simulink model "DEM_testbench_DACerrors"  (Simulink 8.1)
settings: Solver=FixedStepDiscrete  StartTime=0.0  StopTime=60e-3  RelTol=1e-3
values from neighbouring files (symbols this model uses):
  dem_dcin = 1    [init_DAC_3ele.m]    (also in init_DAC_8ele.m)
  dem_select = 4    [init_DAC_3ele.m]    (also in init_DAC_8ele.m)
  dem_sinamp = 2    [init_DAC_3ele.m]    (also in init_DAC_8ele.m = 7)
  dem_sinfreq = 4882.8125    [init_DAC_3ele.m]    (also in init_DAC_8ele.m)
undefined symbols (not defined in the file or in its folder): DACctrl, Fs
libraries: simulink x4, dspsigops x3, dspsrcs4 x2
settings Model: Creator=amyles  LastModifiedBy=amyles
settings DataIOCC: MaxDataPoints=50000
settings DebuggingCC: ParameterPrecisionLossMsg=none  StrictBusMsg=Warning
settings SFSimCC: SimParseCustomCode=off

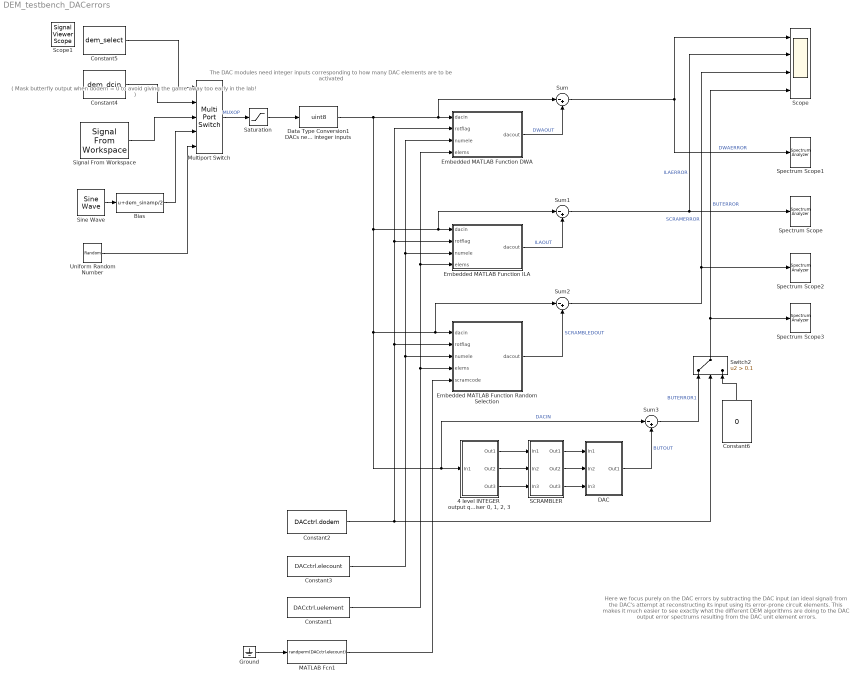
== system DEM_testbench_DACerrors ==
  note: The DAC modules need integer
      | inputs corresponding to how many
      | DAC elements are to be activated
  note: Here we focus purely on the DAC errors by
      | subtracting the DAC input (an ideal signal) from the
      | DAC's attempt at reconstructing its input using its
      | error-prone circuit elements.
      |
      | This makes it much easier to see exactly what the different
      | DEM algorithms are doing to the DAC output error
      | spectrums resulting from the DAC unit element errors.
  note: ( Mask butterfly output when dodem = 0
      | to avoid giving the game away too early
      | in the lab! )
  "4 level INTEGER  output quantiser 0, 1, 2, 3" : Subsystem
  Bias : Bias  Bias=dem_sinamp/2
  Constant1 : Constant  Value=DACctrl.uelement  SampleTime=1/Fs
  Constant2 : Constant  Value=DACctrl.dodem  SampleTime=1/Fs
  Constant3 : Constant  Value=DACctrl.elecount  SampleTime=1/Fs
  Constant4 : Constant  Value=dem_dcin  SampleTime=1/Fs
  Constant5 : Constant  Value=dem_select  SampleTime=1/Fs
  Constant6 : Constant  Value=0  SampleTime=1/Fs
  DAC : Subsystem
  Data Type Conversion1 DACs need integer inputs : DataTypeConversion  OutDataTypeStr=uint8  RndMeth=Nearest
  Embedded MATLAB Function DWA : MATLAB Function  TreatAsAtomicUnit=on
  Embedded MATLAB Function ILA : MATLAB Function  TreatAsAtomicUnit=on
  Embedded MATLAB Function Random Selection : MATLAB Function  TreatAsAtomicUnit=on
  Ground : Ground
  MATLAB Fcn1 : MATLABFcn  MATLABFcn=randperm(DACctrl.elecount)  SampleTime=1/Fs
  Multiport Switch : MultiPortSwitch  Inputs=4
  SCRAMBLER : Subsystem
  Saturation : Saturate  UpperLimit=DACctrl.elecount  LowerLimit=0
  Scope : Scope  NumInputPorts=4
      settings: YMin=-0.04~-5~-5~-5  YMax=0.04~5~5~5
  Signal From Workspace : dspsrcs4/Signal From Workspace  X=[1 1 2]  Ts=1/Fs  nsamps=1  OutputAfterFinalValue=Cyclic repetition  ignoreOrWarnInputAndFrameLengths=off
  Sine Wave : dspsrcs4/Sine Wave  Amplitude=dem_sinamp/2  Frequency=dem_sinfreq  Phase=0  SampleMode=Discrete  OutComplex=Real  CompMethod=Trigonometric fcn  TableSize=Speed  SampleTime=1/Fs  SamplesPerFrame=1  ResetState=Restart at time zero  dataType=double  wordLen=16  udDataType=sfix(16)  fracBitsMode=Best precision  numFracBits=15  OutDataTypeStr=double  LastOutDataTypeStr=double
  Spectrum Scope{,1..3} (4 alike) : SpectrumAnalyzer
      settings: CopyFcn=scopeextensions.ScopeBlock.callback(gcbh, 'onBlockCopy', gcbh);  DeleteFcn=scopeextensions.ScopeBlock.callback(gcbh, 'onBlockDelete');  PreSaveFcn=scopeextensions.ScopeBlock.callback(gcbh, 'onModelSave');  NameChangeFcn=scopeextensions.ScopeBlock.callback(gcbh, 'onBlockRename');  CloseFcn=scopeextensions.ScopeBlock.callback(gcbh, 'onBlockClose');  PreDeleteFcn=scopeextensions.ScopeBlock.callback(gcbh, 'onBlockPreDelete');
  Sum{,1..3} (4 alike) : Sum  Inputs=|-+
  Switch2 : Switch  Criteria=u2 > Threshold  Threshold=0.1
  Uniform Random Number : UniformRandomNumber  Minimum=0  Maximum=DACctrl.elecount  SampleTime=1/Fs
  Scope1 : SignalViewerScope  IOType=viewer  NumInputPorts=2  ZoomMode=xonly  RefreshTime=0.035000
      settings: YMin=0~0  YMax=3~3
  wires:
  Constant5/1 -> Multiport Switch/1
  Signal From Workspace/1 -> Multiport Switch/3
  Sine Wave/1 -> Bias/1
  Multiport Switch/1 -> Saturation/1  "MUXOP"
  Data Type Conversion1 DACs need integer inputs/1 -> Embedded MATLAB Function ILA/1(dacin), Sum1/1, Embedded MATLAB Function Random Selection/1(dacin), Sum2/1, Sum3/1, "4 level INTEGER  output quantiser 0, 1, 2, 3"/1(In1), Embedded MATLAB Function DWA/1(dacin), Sum/1  "DACIN"
  Saturation/1 -> Data Type Conversion1 DACs need integer inputs/1
  Bias/1 -> Multiport Switch/4
  Uniform Random Number/1 -> Multiport Switch/5
  Constant4/1 -> Multiport Switch/2
  Constant2/1 -> Embedded MATLAB Function DWA/2(rotflag), Embedded MATLAB Function ILA/2(rotflag), Embedded MATLAB Function Random Selection/2(rotflag), Switch2/2
  Constant3/1 -> Embedded MATLAB Function DWA/3(numele), Embedded MATLAB Function ILA/3(numele), Embedded MATLAB Function Random Selection/3(numele)
  Constant1/1 -> Embedded MATLAB Function DWA/4(elems), Embedded MATLAB Function ILA/4(elems), Embedded MATLAB Function Random Selection/4(elems)
  Embedded MATLAB Function DWA/1(dacout) -> Sum/2  "DWAOUT"
  Embedded MATLAB Function ILA/1(dacout) -> Sum1/2  "ILAOUT"
  Embedded MATLAB Function Random Selection/1(dacout) -> Sum2/2  "SCRAMBLEDOUT"
  Sum/1 -> Scope/1, Spectrum Scope1/1  "DWAERROR"
  Sum1/1 -> Scope/2, Spectrum Scope/1  "ILAERROR"
  Sum2/1 -> Spectrum Scope2/1, Scope/3  "SCRAMERROR"
  MATLAB Fcn1/1 -> Embedded MATLAB Function Random Selection/5(scramcode)
  Ground/1 -> MATLAB Fcn1/1
  "4 level INTEGER  output quantiser 0, 1, 2, 3"/1(Out1) -> SCRAMBLER/1(In1)
  "4 level INTEGER  output quantiser 0, 1, 2, 3"/2(Out2) -> SCRAMBLER/2(In2)
  "4 level INTEGER  output quantiser 0, 1, 2, 3"/3(Out3) -> SCRAMBLER/3(In3)
  SCRAMBLER/1(Out1) -> DAC/1(In1)
  SCRAMBLER/2(Out2) -> DAC/2(In2)
  SCRAMBLER/3(Out3) -> DAC/3(In3)
  DAC/1(Out1) -> Sum3/2  "BUTOUT"
  Switch2/1 -> Spectrum Scope3/1, Scope/4  "BUTERROR"
  Constant6/1 -> Switch2/3
  Sum3/1 -> Switch2/1  "BUTERROR1"

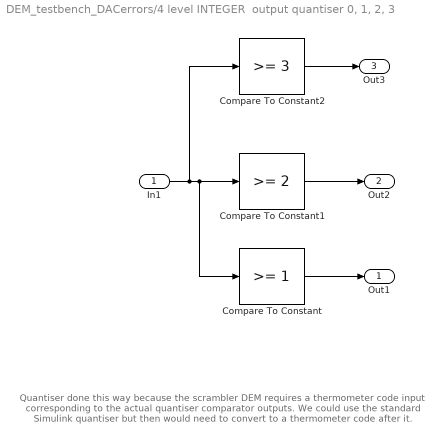
== system DEM_testbench_DACerrors/4 level INTEGER  output quantiser 0, 1, 2, 3 ==
  note: Quantiser done this way because the scrambler DEM
      | requires a thermometer code input corresponding to
      | the actual quantiser comparator outputs. We could use the
      | standard Simulink quantiser but then would need to convert
      | to a thermometer code after it.
  In1 : Inport
  Compare To Constant : simulink/Logic and Bit Operations/Compare To Constant  relop=>=  const=1  OutDataTypeStr=uint8
  Compare To Constant1 : simulink/Logic and Bit Operations/Compare To Constant  relop=>=  const=2  OutDataTypeStr=uint8
  Compare To Constant2 : simulink/Logic and Bit Operations/Compare To Constant  relop=>=  const=3  OutDataTypeStr=uint8
  Out1 : Outport
  Out2 : Outport  Port=2
  Out3 : Outport  Port=3
  wires:
  Compare To Constant2/1 -> Out3/1
  Compare To Constant1/1 -> Out2/1
  Compare To Constant/1 -> Out1/1
  In1/1 -> Compare To Constant2/1, Compare To Constant1/1, Compare To Constant/1

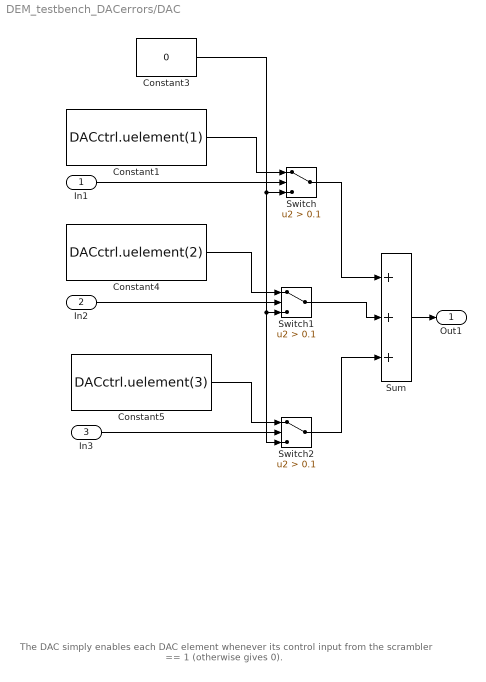
== system DEM_testbench_DACerrors/DAC ==
  note: The DAC simply enables each DAC element whenever its control
      | input from the scrambler == 1 (otherwise gives 0).
  In1 : Inport
  In2 : Inport  Port=2
  In3 : Inport  Port=3
  Constant1 : Constant  Value=DACctrl.uelement(1)  SampleTime=1/Fs
  Constant3 : Constant  Value=0  SampleTime=1/Fs
  Constant4 : Constant  Value=DACctrl.uelement(2)  SampleTime=1/Fs
  Constant5 : Constant  Value=DACctrl.uelement(3)  SampleTime=1/Fs
  Sum : Sum  Inputs=+++
  Switch : Switch  Criteria=u2 > Threshold  Threshold=0.1
  Switch1 : Switch  Criteria=u2 > Threshold  Threshold=0.1
  Switch2 : Switch  Criteria=u2 > Threshold  Threshold=0.1
  Out1 : Outport
  wires:
  Constant5/1 -> Switch2/1
  Constant4/1 -> Switch1/1
  Constant1/1 -> Switch/1
  Constant3/1 -> Switch2/3, Switch1/3, Switch/3
  In3/1 -> Switch2/2
  Sum/1 -> Out1/1
  In2/1 -> Switch1/2
  In1/1 -> Switch/2
  Switch2/1 -> Sum/3
  Switch1/1 -> Sum/2
  Switch/1 -> Sum/1

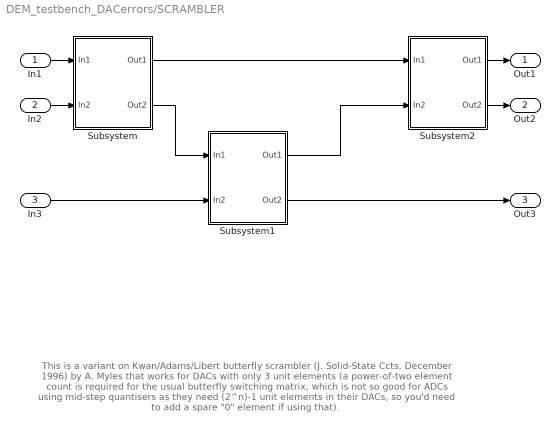
== system DEM_testbench_DACerrors/SCRAMBLER ==
  note: This is a variant on
      |
      | Kwan/Adams/Libert butterfly scrambler
      | (J. Solid-State Ccts. December 1996)
      |
      | by A. Myles that works for DACs with only 3 unit elements
      | (a power-of-two element count is required for the usual
      | butterfly switching matrix, which is not so good for
      | ADCs using mid-step quantisers as they need
      | (2^n)-1 unit elements in their DACs, so you'd need to
      | add a spare "0" element if using that).
  In1 : Inport
  In2 : Inport  Port=2
  In3 : Inport  Port=3
  Subsystem : Subsystem
  Subsystem1 : Subsystem
      settings: AttributesFormatString=Non-standard\nswitching block
  Subsystem2 : Subsystem
  Out1 : Outport
  Out2 : Outport  Port=2
  Out3 : Outport  Port=3
  wires:
  Subsystem1/1(Out1) -> Subsystem2/2(In2)
  Subsystem/2(Out2) -> Subsystem1/1(In1)
  Subsystem1/2(Out2) -> Out3/1
  In3/1 -> Subsystem1/2(In2)
  Subsystem2/2(Out2) -> Out2/1
  In2/1 -> Subsystem/2(In2)
  Subsystem2/1(Out1) -> Out1/1
  In1/1 -> Subsystem/1(In1)
  Subsystem/1(Out1) -> Subsystem2/1(In1)

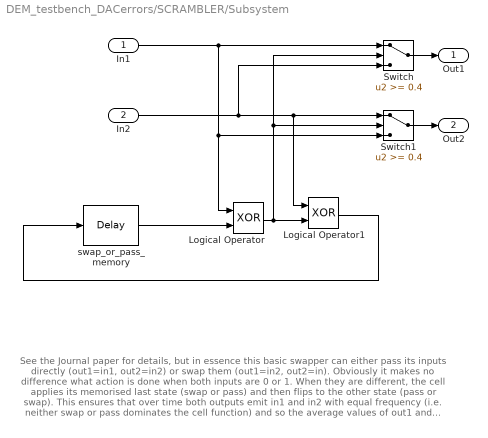
== system DEM_testbench_DACerrors/SCRAMBLER/Subsystem ==
  note: See the Journal paper for details, but in essence this basic swapper
      | can either pass its inputs directly (out1=in1, out2=in2) or swap
      | them (out1=in2, out2=in). Obviously it makes no difference what
      | action is done when both inputs are 0 or 1. When they are different,
      | the cell applies its memorised last state (swap or pass) and then flips
      | to the other state (pass or swap). This ensures that over time
      | both outputs emit in1 and in2 with equal frequency (i.e. neither
      | swap or pass dominates the cell function) and so the average values
      | of out1 and out2 are both (in1+in2)/2.
  In1 : Inport
  In2 : Inport  Port=2
  Logical Operator : Logic  Operator=XOR  AllPortsSameDT=off  OutDataTypeStr=boolean
  Logical Operator1 : Logic  Operator=XOR  AllPortsSameDT=off  OutDataTypeStr=boolean
  Switch : Switch  Threshold=0.4
  Switch1 : Switch  Threshold=0.4
  swap_or_pass_memory : dspsigops/Delay  InputProcessing=Columns as channels (frame based)  dly_unit=Samples  delay=1  ic_detail=off  dif_ic_for_ch=off  dif_ic_for_dly=off  ic=0  reset_popup=None
  Out1 : Outport
  Out2 : Outport  Port=2
  wires:
  Switch1/1 -> Out2/1
  Switch/1 -> Out1/1
  swap_or_pass_memory/1 -> Logical Operator/2
  Logical Operator1/1 -> swap_or_pass_memory/1
  Logical Operator/1 -> Logical Operator1/2, Switch1/2, Switch/2
  In2/1 -> Switch/3, Switch1/1, Logical Operator1/1
  In1/1 -> Switch/1, Switch1/3, Logical Operator/1

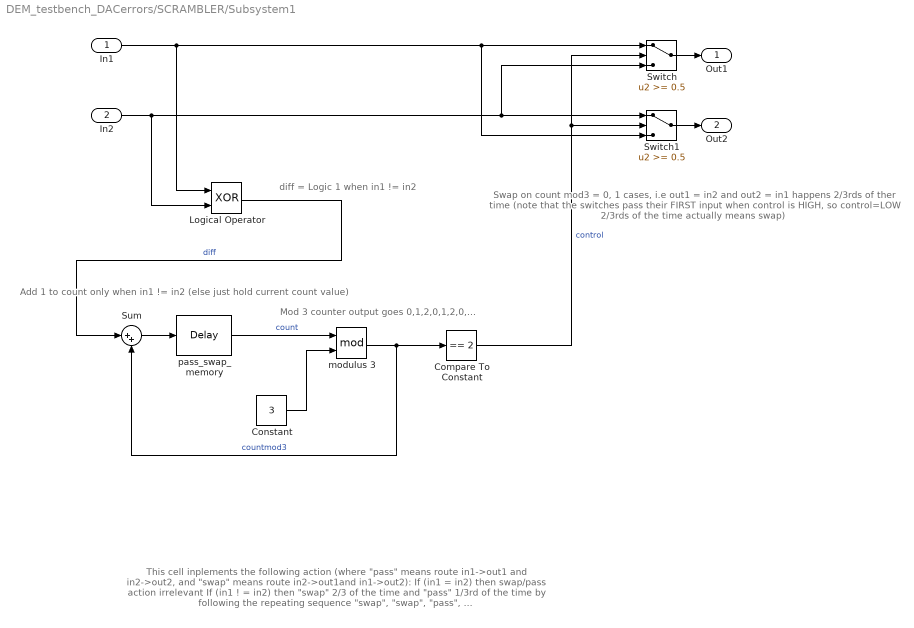
== system DEM_testbench_DACerrors/SCRAMBLER/Subsystem1 ==
  note: Swap on count mod3 = 0, 1 cases,
      | i.e out1 = in2 and out2 = in1
      | happens 2/3rds of ther time
      | (note that the switches pass
      | their FIRST input when control
      | is HIGH, so control=LOW 2/3rds
      | of the time actually means swap)
  note: Mod 3 counter output goes 0,1,2,0,1,2,0,...
  note: diff = Logic 1 when in1 != in2
  note: This cell inplements the following action
      | (where "pass" means route in1->out1 and in2->out2,
      | and "swap" means route in2->out1and in1->out2):
      |
      | If (in1 = in2) then swap/pass action irrelevant
      |
      | If (in1 ! = in2) then "swap" 2/3 of the time and "pass"
      | 1/3rd of the time by following the repeating sequence
      | "swap", "swap", "pass", ...
  note: Add 1 to count only when in1 != in2
      | (else just hold current count value)
  In1 : Inport
  In2 : Inport  Port=2
  Compare To Constant : simulink/Logic and Bit Operations/Compare To Constant  relop===  const=2  OutDataTypeStr=boolean
  Constant : Constant  Value=3
  Logical Operator : Logic  Operator=XOR  AllPortsSameDT=off  OutDataTypeStr=boolean
  Sum : Sum  Inputs=|++
  Switch : Switch  Threshold=0.5
  Switch1 : Switch  Threshold=0.5
  modulus 3 : Math  Operator=mod  SaturateOnIntegerOverflow=on
  pass_swap_memory : dspsigops/Delay  InputProcessing=Columns as channels (frame based)  dly_unit=Samples  delay=1  ic_detail=off  dif_ic_for_ch=off  dif_ic_for_dly=off  ic=0  reset_popup=None
  Out1 : Outport
  Out2 : Outport  Port=2
  wires:
  Compare To Constant/1 -> Switch/2, Switch1/2  "control"
  Sum/1 -> pass_swap_memory/1
  pass_swap_memory/1 -> modulus 3/1  "count"
  modulus 3/1 -> Sum/2, Compare To Constant/1  "countmod3"
  Constant/1 -> modulus 3/2
  Logical Operator/1 -> Sum/1  "diff"
  In1/1 -> Logical Operator/1, Switch1/3, Switch/1
  In2/1 -> Logical Operator/2, Switch1/1, Switch/3
  Switch/1 -> Out1/1
  Switch1/1 -> Out2/1

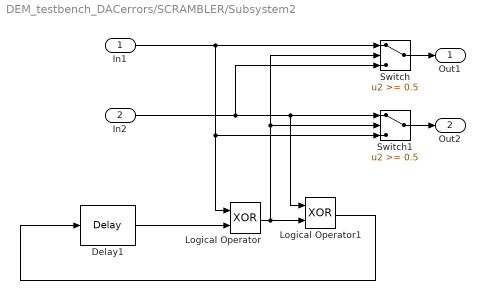
== system DEM_testbench_DACerrors/SCRAMBLER/Subsystem2 ==
  In1 : Inport
  In2 : Inport  Port=2
  Delay1 : dspsigops/Delay  InputProcessing=Columns as channels (frame based)  dly_unit=Samples  delay=1  ic_detail=off  dif_ic_for_ch=off  dif_ic_for_dly=off  ic=0  reset_popup=None
  Logical Operator : Logic  Operator=XOR  AllPortsSameDT=off  OutDataTypeStr=boolean
  Logical Operator1 : Logic  Operator=XOR  AllPortsSameDT=off  OutDataTypeStr=boolean
  Switch : Switch  Threshold=0.5
  Switch1 : Switch  Threshold=0.5
  Out1 : Outport
  Out2 : Outport  Port=2
  wires:
  In1/1 -> Logical Operator/1, Switch1/3, Switch/1
  In2/1 -> Logical Operator1/1, Switch1/1, Switch/3
  Logical Operator/1 -> Switch/2, Switch1/2, Logical Operator1/2
  Logical Operator1/1 -> Delay1/1
  Delay1/1 -> Logical Operator/2
  Switch/1 -> Out1/1
  Switch1/1 -> Out2/1

== matlab function Embedded MATLAB Function ILA ==
  data: dacin input double; dacout output double; rotflag input double; numele input double; elems input double
function dacout = DAC(dacin, rotflag, numele, elems)
%#eml

% This function assumes a MATLAB workspace structures exists called
% DACctrl with contents:
%
% DACctrl.dodem = DEM enable flag, 0 = no ILA, 1 = apply ILA
% DACctrl.elecount = number fo unit elements in the DAC
% DACctrl.uelement(1) = size of first unit element
% ...
% DACctrl.uelement(elecount) = size of last unit element

% ------------------ Begin Copyright notice -----------------------------
%
% COPYRIGHT AND PROPERTY OF DIALOG SEMICONDUCTOR, 2012.
%
% THIS COPYRIGHT NOTICE MUST NOT BE REMOVED OR MODIFIED.
%
% Commerical use is not permitted.
%
% Installation on systems available for use in any way by commercial users
% is not permitted.
%
% Permission for use is granted by Dialog Semiconductor only for the
% purposes of teaching or studying course ELEE11080/PGEE11110 "Sigma
% Delta Data Converters" (or any renamed variant or descendant of
% this course) at the University of Edinburgh.
%
% Personal copying and/or modification is permitted only by students and
% teaching staff of course PGEE11110 solely for the purposes of delivering
% or studying course PGEE11110.
%
% All permissions for use of this or modified copies are revoked upon
% ceasation of teaching duties or completion or de-enrollment for any
% reason from course PGEE11110.
%
% ------------------- End Copyright notice ------------------------------

persistent ila_pointer; % Need a persistent rotator state

dacplus1 = dacin+1; % Quantiser starts at 0, MATLAB array indices at 1...

% static memory cannot be dynamic, so just allocate enough for
% any realistic DAC. Edit this function if you *really* need more
% than 100 DAC elements...

if isempty(ila_pointer)
    ila_pointer = ones(1,100);    % initialise per-code indices
end

if (rotflag == 0)
    ila_pointer(1,dacplus1) = 1;    % reset if not rotating
end

dacout = 0.0;
ipt = ila_pointer(1,dacplus1);
for indx = 1:1:dacin
    dacout = dacout + elems(ipt);
    ipt = mod(ipt, numele) + 1;
% Above line is a faster way of saying...
%     ila_pointer(dacplus1) = ila_pointer(dacplus1) + 1;
%     if (ila_pointer(dacplus1) > numele)
%         ila_pointer(dacplus1) = 1;
%    end
end
ila_pointer(1,dacplus1) = ipt;

end

== matlab function Embedded MATLAB Function DWA ==
  data: dacin input double; dacout output double; rotflag input double; numele input double; elems input double
function dacout = DAC(dacin, rotflag, numele, elems)
%#eml

% This function assumes a MATLAB workspace structures exists called
% DACctrl with contents:
%
% DACctrl.dodem = DEM enable flag, 0 = no DWA, 1 = apply DWA
% DACctrl.elecount = number fo unit elements in the DAC
% DACctrl.uelement(1) = size of first unit element
% ...
% DACctrl.uelement(elecount) = size of last unit element

% ------------------ Begin Copyright notice -----------------------------
%
% COPYRIGHT AND PROPERTY OF DIALOG SEMICONDUCTOR, 2012.
%
% THIS COPYRIGHT NOTICE MUST NOT BE REMOVED OR MODIFIED.
%
% Commerical use is not permitted.
%
% Installation on systems available for use in any way by commercial users
% is not permitted.
%
% Permission for use is granted by Dialog Semiconductor only for the
% purposes of teaching or studying course ELEE11080/PGEE11110 "Sigma
% Delta Data Converters" (or any renamed variant or descendant of
% this course) at the University of Edinburgh.
%
% Personal copying and/or modification is permitted only by students and
% teaching staff of course PGEE11110 solely for the purposes of delivering
% or studying course PGEE11110.
%
% All permissions for use of this or modified copies are revoked upon
% ceasation of teaching duties or completion or de-enrollment for any
% reason from course PGEE11110.
%
% ------------------- End Copyright notice ------------------------------

persistent dwa_pointer; % Need a persistent rotator state

if isempty(dwa_pointer) || (rotflag == 0)
    dwa_pointer = 1;    % initialise or reset if not rotating
end

dacout = 0.0;
for indx = 1:1:dacin
    dacout = dacout + elems(dwa_pointer);
    dwa_pointer = dwa_pointer + 1;
    if (dwa_pointer > numele)
        dwa_pointer = 1;
    end
end

end

== matlab function Embedded MATLAB Function Random Selection ==
  data: dacin input double; dacout output double; rotflag input double; numele input double; elems input double; scramcode input double
function dacout = DAC(dacin, rotflag, numele, elems, scramcode)
%#eml

% This function assumes a MATLAB workspace structures exists called
% DACctrl with contents:
%
% DACctrl.dodem = DEM enable flag, 0 = no scramble, 1 = scramble
% DACctrl.elecount = number fo unit elements in the DAC
% DACctrl.uelement(1) = size of first unit element
% ...
% DACctrl.uelement(elecount) = size of last unit element

%eml.extrinsic('randperm');

% This version allows dynamic resizing of the DAC by moving the randperm
% function call up a level... look how much slower that makes Simulink
% run though!

% ------------------ Begin Copyright notice -----------------------------
%
% COPYRIGHT AND PROPERTY OF DIALOG SEMICONDUCTOR, 2012.
%
% THIS COPYRIGHT NOTICE MUST NOT BE REMOVED OR MODIFIED.
%
% Commerical use is not permitted.
%
% Installation on systems available for use in any way by commercial users
% is not permitted.
%
% Permission for use is granted by Dialog Semiconductor only for the
% purposes of teaching or studying course ELEE11080/PGEE11110 "Sigma
% Delta Data Converters" (or any renamed variant or descendant of
% this course) at the University of Edinburgh.
%
% Personal copying and/or modification is permitted only by students and
% teaching staff of course PGEE11110 solely for the purposes of delivering
% or studying course PGEE11110.
%
% All permissions for use of this or modified copies are revoked upon
% ceasation of teaching duties or completion or de-enrollment for any
% reason from course PGEE11110.
%
% ------------------- End Copyright notice ------------------------------

if (rotflag == 0)
    dacout = sum(elems(1:dacin));
else
    dacout = sum(elems(scramcode(1:dacin)));
end

end
